simulink model "sim_tiso"  (R2024b)
settings: Solver=VariableStepAuto  StartTime=0.0  StopTime=10.0  RelTol=1e-3
values from neighbouring files (symbols this model uses):
  A = [A1', [A2; zeros(1,5)]]    [julio1.m]    (also in tiso1_1.m)
  D = A1'    [julio1.m]    (also in tiso1_1.m)
  H = zeros(1,N)    [julio1.m]    (also in tiso1_1.m)
undefined symbols (not defined in the file or in its folder): B, I1, K, kr, Kur
libraries: cstblocks x1
settings Model: Creator=room2  LastModifiedBy=room2

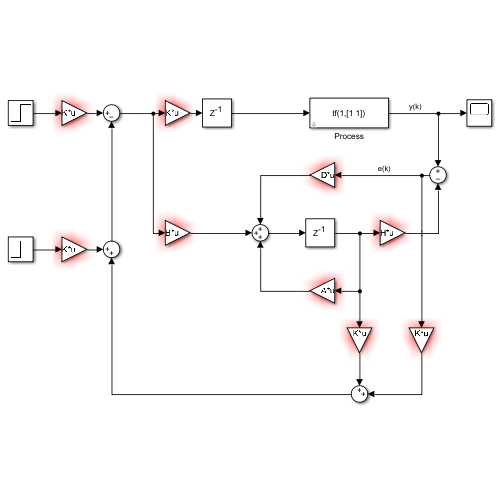
[thumbnail: Simulink's stored preview of the top-level diagram]
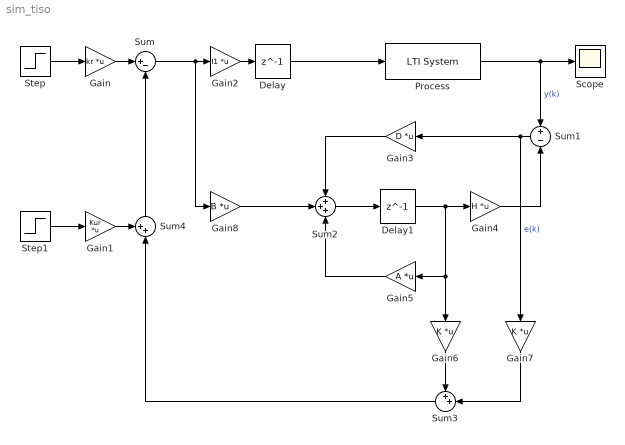
== system sim_tiso ==
  Delay : Delay  DelayLength=1
  Delay1 : Delay  DelayLength=1
  Gain : Gain  Gain=kr  Multiplication=Matrix(K*u)
  Gain1 : Gain  Gain=Kur  Multiplication=Matrix(K*u)
  Gain2 : Gain  Gain=I1  Multiplication=Matrix(K*u)
  Gain3 : Gain  Gain=D  Multiplication=Matrix(K*u)
  Gain4 : Gain  Gain=H  Multiplication=Matrix(K*u)
  Gain5 : Gain  Gain=A  Multiplication=Matrix(K*u)
  Gain6 : Gain  Gain=K  Multiplication=Matrix(K*u)
  Gain7 : Gain  Gain=K  Multiplication=Matrix(K*u)
  Gain8 : Gain  Gain=B  Multiplication=Matrix(K*u)
  Process : cstblocks/LTI System  sys=tf(1,[1 1])  IC=[]  PadeOrder=0
  Scope : Scope
  Step : Step  SampleTime=0
  Step1 : Step  SampleTime=0
  Sum : Sum  Inputs=|+-
  Sum1 : Sum  Inputs=+-
  Sum2 : Sum  Inputs=+++
  Sum3 : Sum  Inputs=++|
  Sum4 : Sum  Inputs=++|
  wires:
  Step/1 -> Gain/1
  Step1/1 -> Gain1/1
  Gain/1 -> Sum/1
  Sum/1 -> Gain8/1, Gain2/1
  Gain2/1 -> Delay/1
  Delay/1 -> Process/1
  Process/1 -> Sum1/1, Scope/1  "y(k)"
  Sum1/1 -> Gain7/1, Gain3/1  "e(k)"
  Delay1/1 -> Gain5/1, Gain6/1, Gain4/1
  Gain4/1 -> Sum1/2
  Gain5/1 -> Sum2/3
  Gain3/1 -> Sum2/1
  Gain8/1 -> Sum2/2
  Sum2/1 -> Delay1/1
  Gain6/1 -> Sum3/1
  Gain7/1 -> Sum3/2
  Gain1/1 -> Sum4/1
  Sum3/1 -> Sum4/2
  Sum4/1 -> Sum/2
